simulink model "Model_3"  (R2020b)
settings: Solver=VariableStepAuto  StartTime=0.0  StopTime=10.0  RelTol=1e-3
settings Model: Creator=Akarsh  LastModifiedBy=Akarsh

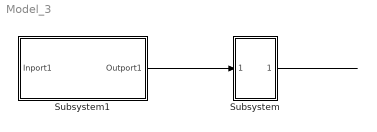
== system Model_3 ==
  Subsystem : Subsystem
  Subsystem1 : Subsystem
  wires:
  Subsystem1/1(Outport1) -> Subsystem/1(In1)
  Subsystem/1(Out1) -> ?
  ? -> Subsystem1/1(Inport1)

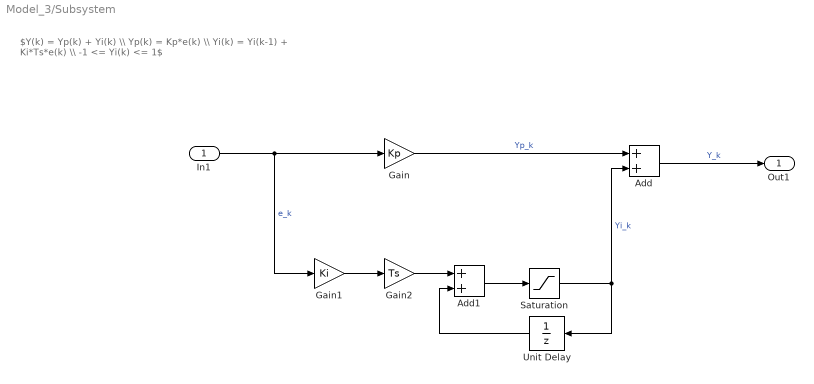
== system Model_3/Subsystem ==
  note: $Y(k) = Yp(k) + Yi(k) \\ Yp(k) = Kp*e(k) \\ Yi(k) = Yi(k-1) + Ki*Ts*e(k) \\ -1 <= Yi(k) <= 1$
  In1 : Inport  OutDataTypeStr=double  PortDimensions=1  SampleTime=0
  Add : Sum
  Add1 : Sum
  Gain : Gain  Gain=Kp  mask{Kp=200, Parameter2=200}
  Gain1 : Gain  Gain=Ki  mask{Ki=120}
  Gain2 : Gain  Gain=Ts  mask{Ts=0.01}
  Saturation : Saturate  UpperLimit=1  LowerLimit=-1
  Unit Delay : UnitDelay  SampleTime=-1  HasFrameUpgradeWarning=on
  Out1 : Outport  OutDataTypeStr=double  PortDimensions=1  SampleTime=0
  wires:
  In1/1 -> Gain/1, Gain1/1  "e_k"
  Unit Delay/1 -> Add1/2
  Saturation/1 -> Unit Delay/1, Add/2  "Yi_k"
  Gain/1 -> Add/1  "Yp_k"
  Add/1 -> Out1/1  "Y_k"
  Gain1/1 -> Gain2/1
  Gain2/1 -> Add1/1
  Add1/1 -> Saturation/1

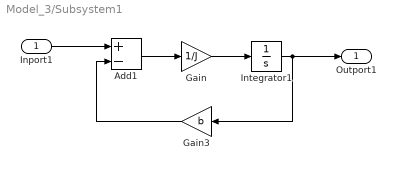
== system Model_3/Subsystem1 ==
  Inport1 : Inport
  Add1 : Sum  Inputs=+-
  Gain : Gain  Gain=1/J  mask{J=100}
  Gain3 : Gain  Gain=b  mask{b=20, Parameter2=0}
  Integrator1 : Integrator
  Outport1 : Outport
  wires:
  Add1/1 -> Gain/1
  Integrator1/1 -> Outport1/1, Gain3/1
  Gain/1 -> Integrator1/1
  Gain3/1 -> Add1/2
  Inport1/1 -> Add1/1
